simulink model "working_simulink_model"  (R2020b)
settings: Solver=ode3  StartTime=0.0  StopTime=10.0  FixedStep=0.001  RelTol=1e-3
undefined symbols (not defined in the file): DiscIntNeverNeededParam, National_Instruments, PCIe, sens, Ts
libraries: sldrtlib x3, simulink x2
settings Model: Creator=controlsystemsuser  LastModifiedBy=controlsystemsuser
settings DataIOCC: ReturnWorkspaceOutputs=off
settings RTWCC: Description=Simulink Desktop Real-Time  SystemTargetFile=sldrt.tlc  TemplateMakefile=sldrt.tmf  RTWCompilerOptimization=on
settings CodeAppCC: MaxIdLength=95
settings SimulinkDesktopRealTimeCC: TargetPreCompLibLocation=C:\Program Files\MATLAB\R2020b\toolbox\sldrt\lib\win64

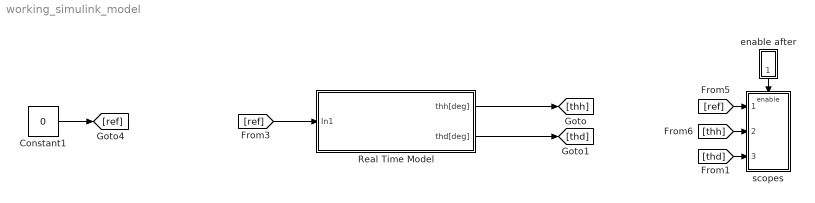
== system working_simulink_model ==
  Constant1 : Constant  Value=0
  Real Time Model : Subsystem
  enable after : Subsystem
  scopes : Subsystem
  wires:
  enable after/1(1.0 s) -> scopes/Enable
  [thd] -> scopes/3(thd[deg])
  [thh] -> scopes/2(thh[deg])
  [ref] -> scopes/1(ref[deg])
  Real Time Model/2(thd[deg]) -> [thd]
  Real Time Model/1(thh[deg]) -> [thh]
  Constant1/1 -> [ref]
  [ref] -> Real Time Model/1(In1)

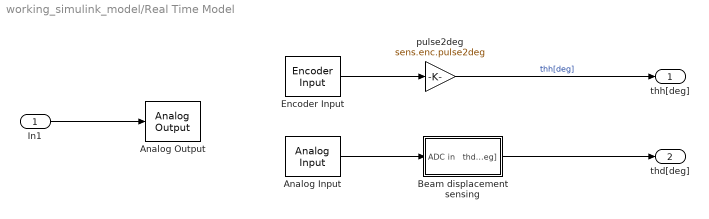
== system working_simulink_model/Real Time Model ==
  In1 : Inport
  Analog Input : sldrtlib/Analog Input  SampleTime=0.001  MaxMissedTicks=10  ShowMissedTicks=off  YieldWhenWaiting=off  DrvName=National_Instruments/PCIe-6321  DrvAddress=4294967295  DrvOptions=[0 0 0 2 0 0 0]  Channels=[3,4]  RangeMode=1  VoltRange=2  DataType=1
      settings: AttributesFormatString=National Instruments\nPCIe-6321 [auto]
  Analog Output : sldrtlib/Analog Output  SampleTime=0.001  MaxMissedTicks=10  ShowMissedTicks=off  YieldWhenWaiting=off  DrvName=National_Instruments/PCIe-6321  DrvAddress=4294967295  DrvOptions=[0 0 0 2 0 0 0]  Channels=1  RangeMode=1  VoltRange=1  InitialValue=0  FinalValue=0
      settings: AttributesFormatString=National Instruments\nPCIe-6321 [auto]
  Beam displacement sensing : Subsystem
  Encoder Input : sldrtlib/Encoder Input  SampleTime=0.001  MaxMissedTicks=10  ShowMissedTicks=off  YieldWhenWaiting=off  DrvName=National_Instruments/PCIe-6321  DrvAddress=4294967295  DrvOptions=[0 0 0 2 0 0 0]  Channels=1  QuadMode=3  IndexPulse=1  InputFilter=Inf  DataType=1
      settings: AttributesFormatString=National Instruments\nPCIe-6321 [auto]
  pulse2deg : Gain  Gain=sens.enc.pulse2deg
  thh[deg] : Outport
  thd[deg] : Outport  Port=2
  wires:
  Encoder Input/1 -> pulse2deg/1
  Beam displacement sensing/1(thd[deg]) -> thd[deg]/1
  Analog Input/1 -> Beam displacement sensing/1(ADC in)
  pulse2deg/1 -> thh[deg]/1  "thh[deg]"
  In1/1 -> Analog Output/1

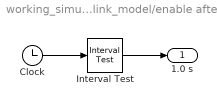
== system working_simulink_model/enable after ==
  Clock : Clock
  Interval Test : simulink/Logic and Bit Operations/Interval Test  IntervalClosedRight=on  uplimit=inf  IntervalClosedLeft=on  lowlimit=1  OutDataTypeStr=boolean
  1.0 s : Outport
  wires:
  Interval Test/1 -> 1.0 s/1
  Clock/1 -> Interval Test/1

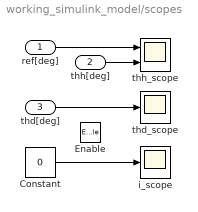
== system working_simulink_model/scopes ==
  ref[deg] : Inport
  thh[deg] : Inport  Port=2
  thd[deg] : Inport  Port=3
  Enable : EnablePort
  Constant : Constant  Value=0
  i_scope : Scope
  thd_scope : Scope
  thh_scope : Scope  NumInputPorts=2
  wires:
  thd[deg]/1 -> thd_scope/1
  Constant/1 -> i_scope/1
  thh[deg]/1 -> thh_scope/2
  ref[deg]/1 -> thh_scope/1

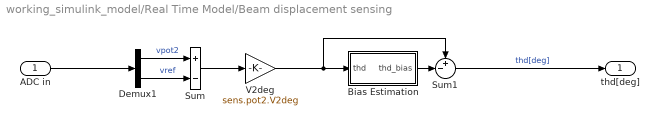
== system working_simulink_model/Real Time Model/Beam displacement sensing ==
  ADC in : Inport
  Bias Estimation : Subsystem
  Demux1 : Demux  Outputs=2
  Sum : Sum  Inputs=+-
  Sum1 : Sum  Inputs=+-|
  V2deg : Gain  Gain=sens.pot2.V2deg
  thd[deg] : Outport
  wires:
  Bias Estimation/1(thd_bias) -> Sum1/2
  Sum/1 -> V2deg/1
  Demux1/1 -> Sum/1  "vpot2"
  Demux1/2 -> Sum/2  "vref"
  Sum1/1 -> thd[deg]/1  "thd[deg]"
  V2deg/1 -> Sum1/1, Bias Estimation/1(thd)
  ADC in/1 -> Demux1/1

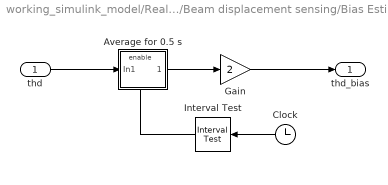
== system working_simulink_model/Real Time Model/Beam displacement sensing/Bias Estimation ==
  thd : Inport
  Average for 0.5 s : Subsystem
  Clock : Clock
  Gain : Gain  Gain=2
  Interval Test : simulink/Logic and Bit Operations/Interval Test  IntervalClosedRight=on  uplimit=0.7  IntervalClosedLeft=on  lowlimit=0.2  OutDataTypeStr=boolean
  thd_bias : Outport
  wires:
  Interval Test/1 -> Average for 0.5 s/Enable
  thd/1 -> Average for 0.5 s/1(In1)
  Clock/1 -> Interval Test/1
  Average for 0.5 s/1(Out1) -> Gain/1
  Gain/1 -> thd_bias/1

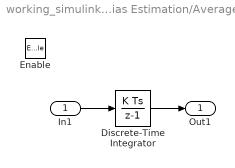
== system working_simulink_model/Real Time Model/Beam displacement sensing/Bias Estimation/Average for 0.5 s ==
  In1 : Inport
  Enable : EnablePort
  Discrete-Time Integrator : DiscreteIntegrator  SampleTime=Ts  ICPrevOutput=DiscIntNeverNeededParam  ICPrevScaledInput=DiscIntNeverNeededParam
  Out1 : Outport
  wires:
  In1/1 -> Discrete-Time Integrator/1
  Discrete-Time Integrator/1 -> Out1/1
